simulink model "ddc_simulink_CRD"  (R2022b)
settings: Solver=VariableStepAuto  StartTime=0.0  StopTime=10.0  RelTol=1e-3
undefined symbols (not defined in the file): Fs, Ts
libraries: dspsrcs4 x1, dspfdesign x1, dsphdlsigops2 x1
settings Model: Creator=caleb  LastModifiedBy=caleb

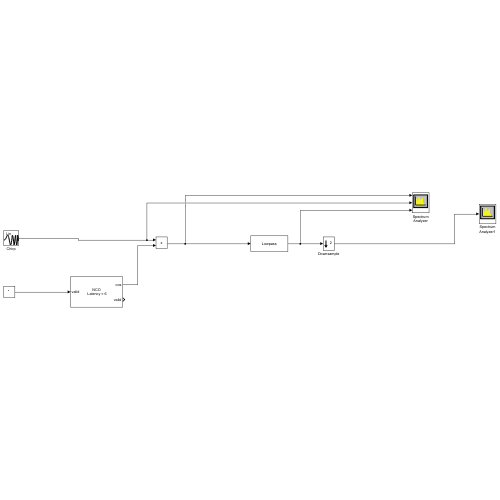
[thumbnail: Simulink's stored preview of the top-level diagram]
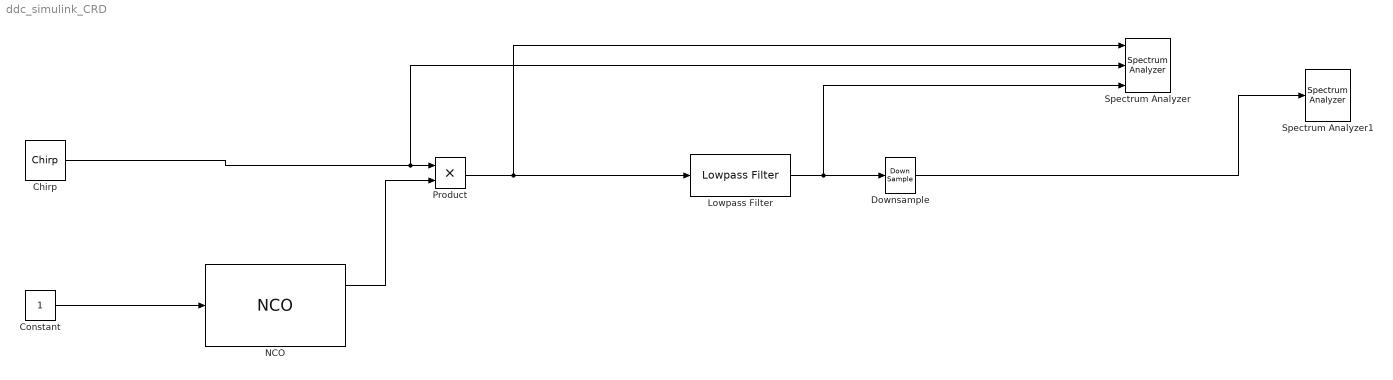
== system ddc_simulink_CRD ==
  Chirp : dspsrcs4/Chirp  sweep=Linear  mode=Unidirectional  f0=10e6  f1=20e6  t1=0.00001998  Tsweep=0.00001998  phase=0  Ts=1/Fs  spf=1  datatype=Double  OutputFrames=off
  Constant : Constant  OutDataTypeStr=boolean  SampleTime=Ts
  Downsample : DownSample  RateOptions=Allow multirate processing
  Lowpass Filter : dspfdesign/Lowpass Filter  FilterType=FIR  DesignForMinimumOrder=off  FilterOrder=96  PassbandFrequency=Fc  StopbandFrequency=Fc  PassbandRipple=0.1  StopbandAttenuation=80  InheritSampleRate=off  SampleRate=Fs  SimulateUsing=Interpreted execution  roundingMode=Floor  coeffsDataTypeStr=fixdt(1,16)
  NCO : dsphdlsigops2/NCO  PhaseIncrementSource=Property  PhaseIncrement=phIncr  PhaseOffsetSource=Property  PhaseOffset=phOff  DitherSource=Property  NumDitherBits=ditherBits  SamplesPerFrame=1  LUTCompress=off  ResetAction=off  Waveform=Cosine  PhasePort=off  SimulateUsing=Code generation  AccumulatorWL=N  PhaseQuantization=on  NumQuantizerAccumulatorBits=Q  OutputDataType=Binary point scaling  OutputWL=16  OutputFL=14
  Product : Product
  Spectrum Analyzer : SpectrumAnalyzer  NumInputPorts=3
  Spectrum Analyzer1 : SpectrumAnalyzer
  wires:
  Constant/1 -> NCO/1
  NCO/1 -> Product/2
  Chirp/1 -> Spectrum Analyzer/2, Product/1
  Product/1 -> Lowpass Filter/1, Spectrum Analyzer/1
  Lowpass Filter/1 -> Downsample/1, Spectrum Analyzer/3
  Downsample/1 -> Spectrum Analyzer1/1
